simulink model "DOOR"  (R2020a)
settings: Solver=FixedStepAuto  StartTime=0.0  StopTime=16  FixedStep=1e-3  RelTol=1e-3  EnableMultiTasking=on
settings Model: ExtModeTrigDuration=5  Creator=theodor  LastModifiedBy=theodor
settings OptimizationCC: EnhancedBackFolding=on  PassReuseOutputArgsAs=Individual arguments  ZeroExternalMemoryAtStartup=off  ZeroInternalMemoryAtStartup=off  MaxStackSize=64  OptimizeBlockOrder=speed  DifferentSizesBufferReuse=on  OptimizationCustomize=off  EfficientTunableParamExpr=on
settings DebuggingCC: ParameterTunabilityLossMsg=error
settings HardwareCC: ProdBitPerPointer=32  ProdBitPerSizeT=32  ProdBitPerPtrDiffT=32  ProdLargestAtomicInteger=Long  ProdLargestAtomicFloat=Double  ProdWordSize=32  ProdHWDeviceType=ARM Compatible->ARM Cortex
settings SFSimCC: MATLABDynamicMemAlloc=off
settings RTWCC: SystemTargetFile=ert.tlc  HardwareBoard=NXP FRDM-K64F  TemplateMakefile=ert_default_tmf  Toolchain=GNU Tools for ARM Embedded Processors
settings CodeAppCC: ForceParamTrailComments=on  IgnoreCustomStorageClasses=off  OperatorAnnotations=on  SimulinkDataObjDesc=on  SFDataObjDesc=on  InsertBlockDesc=on

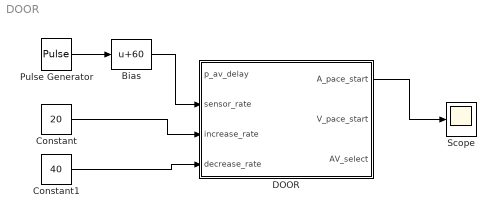
== system DOOR ==
  Bias : Bias  Bias=60
  Constant : Constant  Value=20
  Constant1 : Constant  Value=40
  DOOR : Stateflow chart  TreatAsAtomicUnit=on
  Pulse Generator : DiscretePulseGenerator  PulseType=Time based  Amplitude=60  Period=16  PulseWidth=50
  Scope : Scope
  wires:
  Constant/1 -> DOOR/3(increase_rate)
  Constant1/1 -> DOOR/4(decrease_rate)
  DOOR/1(A_pace_start) -> Scope/1
  Pulse Generator/1 -> Bias/1
  Bias/1 -> DOOR/2(sensor_rate)

== stateflow chart DOOR/DOOR ==
  state INITIAL
    entry:
    current_LRL = sensor_rate;
  state PACE_VENT
    entry:
    V_pace_start = true;
    on after(1, msec):
    V_pace_start = false;
    AV_select = 0;
    exit:
    t = elapsed(sec)
  state PACE_ATR
    entry:
    A_pace_start = true;
    on after(1,msec):
    A_pace_start = false;
    AV_select = 1;
    exit:
    t = t + elapsed(sec)
  (default) -> INITIAL
  INITIAL -> PACE_VENT
  (junction 35) -> (junction 37)
  (junction 37) -> (junction 32)
  (junction 13) -> (junction 35) [order 1] : [current_LRL + increase_rate*t > sensor_rate]{current_LRL = sensor_rate}
  (junction 13) -> (junction 32) [order 2] : {current_LRL = current_LRL + increase_rate*t}
  (junction 32) -> PACE_VENT
  (junction 42) -> (junction 13) [order 2] : [sensor_rate > current_LRL]
  PACE_ATR -> (junction 42) : after(p_av_delay, msec)
  (junction 42) -> (junction 14) [order 1] : [sensor_rate <= current_LRL]
  PACE_VENT -> PACE_ATR : after(60/current_LRL - p_av_delay/1000,sec)
  (junction 24) -> PACE_VENT
  (junction 14) -> (junction 24) [order 2] : {current_LRL = current_LRL - decrease_rate * t}
  (junction 29) -> (junction 24)
  (junction 14) -> (junction 26) [order 1] : [current_LRL - decrease_rate * t  < sensor_rate ]{current_LRL = sensor_rate}
  (junction 26) -> (junction 29)
  data: p_av_delay input; A_pace_start output; V_pace_start output; sensor_rate input; increase_rate input; decrease_rate input; current_LRL local; t local =0; AV_select output
